simulink model "AccTarSel"  (R2018b)
settings: Solver=FixedStepDiscrete  StartTime=0.0  StopTime=inf  FixedStep=0.01  RelTol=1e-3
PostLoadFcn:
  | if any(exist('dsrtsu_mdlpostloadfcn', 'file') ~= 0), dsrtsu_mdlpostloadfcn('Execute', bdroot); end
values from neighbouring files (symbols this model uses):
  P_adtMaxBDC = 1.0    [AccTarSel.sldd]
  P_aFOCApproachIntpAcitve = -0.6    [AccTarSel.sldd]
  P_aFOCApproachIntpEnsure = -1.8    [AccTarSel.sldd]
  P_CutInEnable = 1.0    [AccTarSel.sldd]
  P_dAimMin = 4.5    [AccTarSel.sldd]
  P_dAimMinAVP = 1.5    [AccTarSel.sldd]
  P_dObjDrvOffMax = 5.0    [AccTarSel.sldd]
  P_dObjDrvOffMin = 3.0    [AccTarSel.sldd]
  P_dObjLowHystDecToStop = 4.5    [AccTarSel.sldd]
  P_dObjLowHystDecToStopAVP = 1.5    [AccTarSel.sldd]
  P_dObjUpperHystDecToStop = 5.0    [AccTarSel.sldd]
  P_dResMax = 5.0    [AccTarSel.sldd]
  P_dStandStill = 3.0    [AccTarSel.sldd]
  P_dStandStillMin = 2.0    [AccTarSel.sldd]
  P_dvarYMax4PO = 1.0    [AccTarSel.sldd]
  P_dyCutInThres = 3.6    [AccTarSel.sldd]
  P_facBDCInit = 0.7    [AccTarSel.sldd]
  P_facBDCIterCalc = 0.8    [AccTarSel.sldd]
  P_facFOCNegDiff = 0.3    [AccTarSel.sldd]
  P_facFOCPosDiff = 0.2    [AccTarSel.sldd]
  P_kapHystThres = 0.0005    [AccTarSel.sldd]
  P_PlausIntegDisable = 0.0    [AccTarSel.sldd]
  P_plausMin4PO = 0.5    [AccTarSel.sldd]
  P_probExistMin4PO = 0.8    [AccTarSel.sldd]
  P_StandObjEnable = 0.0    [AccTarSel.sldd]
  P_tAxTrackNegLower = 0.3    [AccTarSel.sldd]
  P_tAxTrackNegUpper = 0.6    [AccTarSel.sldd]
  P_tAxTrackPosLower = 1.0    [AccTarSel.sldd]
  P_tAxTrackPosUpper = 2.0    [AccTarSel.sldd]
  P_tBDCStartFilt = 0.2    [AccTarSel.sldd]
  P_tCSC = 3.5    [AccTarSel.sldd]
  P_tCurvFilt = 0.2    [AccTarSel.sldd]
  P_tCutInFilt = 0.5    [AccTarSel.sldd]
  P_tFiltAxAbsPONegFast = 0.1    [AccTarSel.sldd]
  P_tFiltAxAbsPONegSlow = 0.4    [AccTarSel.sldd]
  P_tFiltAxAbsPOPosFast = 1.2    [AccTarSel.sldd]
  P_tFiltAxAbsPOPosSlow = 2.0    [AccTarSel.sldd]
  P_tFiltAxAbsPOStand = 2.0    [AccTarSel.sldd]
  P_tFiltDAim = 0.1    [AccTarSel.sldd]
  P_tFiltDsd = 0.1    [AccTarSel.sldd]
  P_tFiltSpdLim = 3.0    [AccTarSel.sldd]
  P_tFiltVxAxPOFast = 0.15    [AccTarSel.sldd]
  P_tFiltVxAxPOSlow = 0.25    [AccTarSel.sldd]
  P_tFOCStatAccelFast = 4.0    [AccTarSel.sldd]
  P_tFOCStatAccelSlow = 3.5    [AccTarSel.sldd]
  P_tFOCStatDecelFast = 4.0    [AccTarSel.sldd]
  P_tFOCStatDecelSlow = 3.2    [AccTarSel.sldd]
  P_tMinDrvPhase = 2.0    [AccTarSel.sldd]
  P_tPredObjLeav = 1.2    [AccTarSel.sldd]
  P_tRollingFilt = 0.5    [AccTarSel.sldd]
  P_tRollingFinFilt = 1.0    [AccTarSel.sldd]
  P_tSSCNeg = 4.5    [AccTarSel.sldd]
  P_tSSCPos = 5.5    [AccTarSel.sldd]
  P_tToStop = 5.0    [AccTarSel.sldd]
  P_tToStopInBDC = 6.0    [AccTarSel.sldd]
  P_tToStopTrig = 4.0    [AccTarSel.sldd]
  P_vEgoDecToStop = 3.0    [AccTarSel.sldd]
  P_vEgoLowBDC = 4.0    [AccTarSel.sldd]
  P_vFOCNegDiff = 4.0    [AccTarSel.sldd]
  P_vFOCPosDiff = 5.0    [AccTarSel.sldd]
  P_vFOCStationaryFast = 15.0    [AccTarSel.sldd]
  P_vFOCStationarySlow = 5.0    [AccTarSel.sldd]
  P_vObjDrvOff = 0.5    [AccTarSel.sldd]
  P_vObjLowHystDecToStop = 0.5    [AccTarSel.sldd]
  P_vObjNoStop = 1.0    [AccTarSel.sldd]
  P_vObjReCalc = 1.0    [AccTarSel.sldd]
  P_vObjStop = 0.3    [AccTarSel.sldd]
  P_vObjUpperHystDecToStop = 0.8    [AccTarSel.sldd]
  P_vStandStill = 0.3    [AccTarSel.sldd]
  P_vStandStillHyst = 0.3    [AccTarSel.sldd]
  P_vyCutInThres = 0.5    [AccTarSel.sldd]
libraries: simulink x21, LPFilter x12
(part 7 of 11)

== system AccTarSel/ACC_Control/FollowObjCtrl/FollowObjValid/FOC_MIX ==
  aStat : Inport
  aApprh : Inport  Port=2
  tObjStop : Inport  Port=3
  FOCInfoK1 : Inport  Port=4
  SYS_Info_st : Inport  Port=5
  Bus Creator{,1..3} (4 alike) : BusCreator  Inputs=2
  Bus Selector : BusSelector  OutputSignals=dT
  Bus Selector1 : BusSelector  OutputSignals=FirstCyc,aFOC
  Constant : Constant  Value=3  OutDataTypeStr=single
  Constant1 : Constant  Value=0.1  OutDataTypeStr=single
  Constant2 : Constant  Value=0.4  OutDataTypeStr=single
  Constant4 : Constant  Value=5  OutDataTypeStr=single
  LPFilter : LPFilter/LPFilter  SystemSampleTime=-1
      settings: SourceProductName=CustomLib
  Lookup Table Dynamic : simulink/Lookup Tables/Lookup Table Dynamic  LookUpMeth=Interpolation-Use End Values  OutDataType=fixdt('single')  OutScaling=[]  OutputDataTypeScalingMode=Specify via dialog  OutDataTypeStr=single  DoSatur=off
      settings: SourceProductName=Simulink
  Lookup Table Dynamic1 : simulink/Lookup Tables/Lookup Table Dynamic  LookUpMeth=Interpolation-Use End Values  OutDataType=fixdt('single')  OutScaling=[]  OutputDataTypeScalingMode=Specify via dialog  OutDataTypeStr=single  DoSatur=off
      settings: SourceProductName=Simulink
  Min : MinMax  Inputs=2
  P_aFOCApproachIntpAcitve : Constant  Value=P_aFOCApproachIntpAcitve
  P_aFOCApproachIntpEnsure : Constant  Value=P_aFOCApproachIntpEnsure
  Subsystem : Subsystem
  Switch : Switch  Criteria=u2 > Threshold
  aFocMix : Outport
  wires:
  aApprh/1 -> Min/2, Subsystem/2(In2)
  Bus Creator/1 -> Lookup Table Dynamic/2
  aStat/1 -> Bus Creator1/2, Subsystem/1(In1), Min/1
  Bus Creator1/1 -> Lookup Table Dynamic/3
  P_aFOCApproachIntpEnsure/1 -> Bus Creator/1
  P_aFOCApproachIntpAcitve/1 -> Bus Creator/2
  Min/1 -> Bus Creator1/1, Lookup Table Dynamic/1
  Lookup Table Dynamic/1 -> LPFilter/1, Switch/1
  Switch/1 -> aFocMix/1
  LPFilter/1 -> Switch/3
  SYS_Info_st/1 -> Bus Selector/1
  Constant/1 -> Bus Creator2/1
  Constant4/1 -> Bus Creator2/2
  Constant2/1 -> Bus Creator3/1
  Bus Selector/1 -> LPFilter/2  "<dT>"
  tObjStop/1 -> Lookup Table Dynamic1/1
  Bus Creator2/1 -> Lookup Table Dynamic1/2
  Bus Creator3/1 -> Lookup Table Dynamic1/3
  Lookup Table Dynamic1/1 -> LPFilter/3
  FOCInfoK1/1 -> Bus Selector1/1
  Bus Selector1/1 -> Switch/2  "<FirstCyc>"
  Bus Selector1/2 -> LPFilter/4  "<aFOC>"
  Constant1/1 -> Bus Creator3/2

== system AccTarSel/ACC_Control/FollowObjCtrl/FollowObjValid/If Action Subsystem ==
  In1 : Inport
  Action Port : ActionPort  ActionType=then
  Out1 : Outport
  wires:
  In1/1 -> Out1/1

== system AccTarSel/ACC_Control/FollowObjCtrl/FollowObjValid/If Action Subsystem1 ==
  In1 : Inport
  Action Port : ActionPort  ActionType=else
  Out1 : Outport
  wires:
  In1/1 -> Out1/1

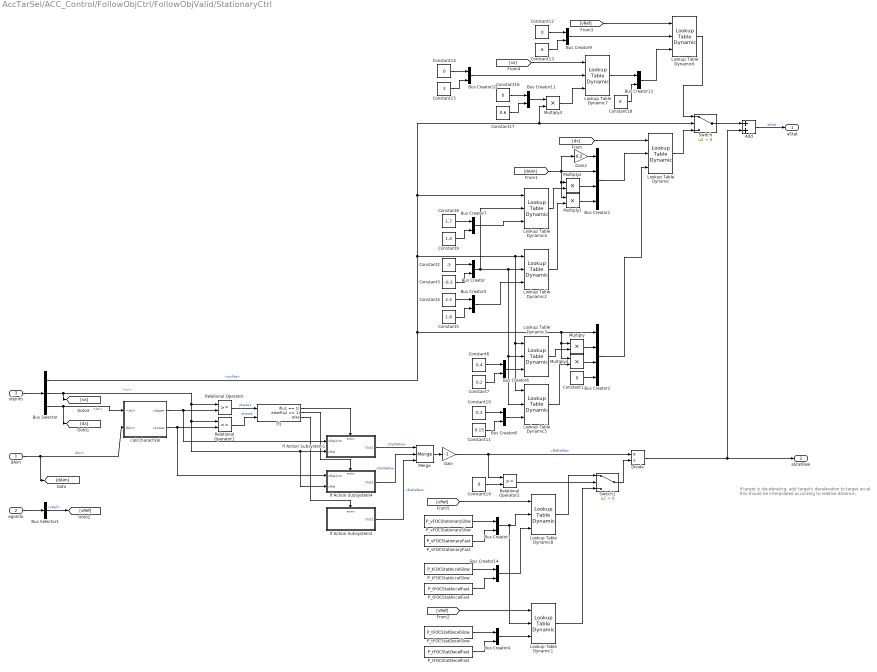
== system AccTarSel/ACC_Control/FollowObjCtrl/FollowObjValid/StationaryCtrl ==
  note: if target is decelerating, add target's deceleration to target accel.
      | this should be interpolated according to relative distance.
  dAim : Inport
  egoInfo : Inport  Port=2
  objInfo : Inport  Port=3
  Add : Sum
  Bus Creator{,3..12,14} (12 alike) : BusCreator  Inputs=2
  Bus Creator1 : BusCreator  Inputs=4
  Bus Creator2 : BusCreator  Inputs=4
  Bus Selector : BusSelector  OutputSignals=axAbs,vx,dx
  Bus Selector1 : BusSelector  OutputSignals=vRef
  Constant{1,12,14,16,18..19} (6 alike) : Constant  Value=0  OutDataTypeStr=single
  Constant10 : Constant  Value=0.3  OutDataTypeStr=single
  Constant11 : Constant  Value=0.15  OutDataTypeStr=single
  Constant13 : Constant  Value=6  OutDataTypeStr=single
  Constant15 : Constant  Value=3  OutDataTypeStr=single
  Constant17 : Constant  Value=0.6  OutDataTypeStr=single
  Constant2 : Constant  Value=-3  OutDataTypeStr=single
  Constant3 : Constant  Value=-0.3  OutDataTypeStr=single
  Constant4 : Constant  Value=2.5  OutDataTypeStr=single
  Constant5 : Constant  Value=1.8  OutDataTypeStr=single
  Constant6 : Constant  Value=0.4  OutDataTypeStr=single
  Constant7 : Constant  Value=0.2  OutDataTypeStr=single
  Constant8 : Constant  Value=1.7  OutDataTypeStr=single
  Constant9 : Constant  Value=1.4  OutDataTypeStr=single
  Divide : Product  Inputs=*/
  Gain : Gain  Gain=-1
  Gain2 : Gain  Gain=0.2
  If Action Subsystem1 : Subsystem  TreatAsAtomicUnit=on
  If Action Subsystem2 : Subsystem  TreatAsAtomicUnit=on
  If Action Subsystem4 : Subsystem  TreatAsAtomicUnit=on
  If1 : If  NumInputs=2  IfExpression=u1 == 1  ElseIfExpressions=u2 == 1
  Lookup Table Dynamic{,1..8} (9 alike) : simulink/Lookup Tables/Lookup Table Dynamic  LookUpMeth=Interpolation-Use End Values  OutDataType=fixdt('single')  OutScaling=[]  OutputDataTypeScalingMode=Specify via dialog  OutDataTypeStr=single  DoSatur=off
      settings: SourceProductName=Simulink
  Merge : Merge  Inputs=3
  Multiply{,1..4} (5 alike) : Product
  P_tFOCStatAccelFast : Constant  Value=P_tFOCStatAccelFast
  P_tFOCStatAccelSlow : Constant  Value=P_tFOCStatAccelSlow
  P_tFOCStatDecelFast : Constant  Value=P_tFOCStatDecelFast
  P_tFOCStatDecelSlow : Constant  Value=P_tFOCStatDecelSlow
  P_vFOCStationaryFast : Constant  Value=P_vFOCStationaryFast
  P_vFOCStationarySlow : Constant  Value=P_vFOCStationarySlow
  Relational Operator : RelationalOperator  OutDataTypeStr=boolean  RndMeth=Simplest
  Relational Operator1 : RelationalOperator  Operator=<=  OutDataTypeStr=boolean  RndMeth=Simplest
  Relational Operator2 : RelationalOperator  OutDataTypeStr=boolean  RndMeth=Simplest
  Switch : Switch  Criteria=u2 > Threshold
  Switch1 : Switch  Criteria=u2 > Threshold
  calcCharactVal : Subsystem
  aStat : Outport
  aStatRaw : Outport  Port=2
  wires:
  objInfo/1 -> Bus Selector/1
  Divide/1 -> Add/2, aStatRaw/1
  Merge/1 -> Gain/1
  dAim/1 -> [dAim], calcCharactVal/2(dAim)  "dAim"
  Bus Selector/3 -> [dx], calcCharactVal/1(<dx>)  "<dx>"
  Bus Selector/2 -> [vx], Relational Operator/1, If Action Subsystem1/2(vRel), If Action Subsystem4/2(vRel), Relational Operator1/1  "<vx>"
  calcCharactVal/2(vLower) -> If Action Subsystem4/1(vRelAim), Relational Operator1/2
  Relational Operator/1 -> If1/1  "phase1"
  Relational Operator1/1 -> If1/2  "phase2"
  If1/1 -> If Action Subsystem1/Action
  If1/2 -> If Action Subsystem4/Action
  If1/3 -> If Action Subsystem2/Action
  If Action Subsystem1/1(Out1) -> Merge/1  "vDeltaRaw"
  If Action Subsystem4/1(Out1) -> Merge/2  "vDeltaRaw"
  If Action Subsystem2/1(Out1) -> Merge/3  "vDeltaRaw"
  Bus Selector/1 -> Lookup Table Dynamic5/1, Lookup Table Dynamic3/1, Lookup Table Dynamic2/1, Lookup Table Dynamic4/1, Switch/2, Multiply3/2, Multiply4/1, Multiply/1, Bus Creator2/1  "<axAbs>"
  calcCharactVal/1(vUpper) -> If Action Subsystem1/1(vRelAim), Relational Operator/2
  Gain/1 -> Relational Operator2/1, Divide/1  "vDeltaRaw"
  [dx] -> Lookup Table Dynamic/1
  Gain2/1 -> Bus Creator1/1
  [dAim] -> Multiply2/1, Multiply1/1, Bus Creator1/2, Gain2/1
  Bus Creator2/1 -> Lookup Table Dynamic/3
  Bus Creator1/1 -> Lookup Table Dynamic/2
  egoInfo/1 -> Bus Selector1/1
  Bus Selector1/1 -> [vRef]  "<vRef>"
  [vRef] -> Lookup Table Dynamic1/1
  P_vFOCStationarySlow/1 -> Bus Creator3/1
  P_vFOCStationaryFast/1 -> Bus Creator3/2
  Bus Creator4/1 -> Lookup Table Dynamic1/3
  Switch/1 -> Add/1
  Add/1 -> aStat/1  "aStat"
  Multiply1/1 -> Bus Creator1/4
  Constant1/1 -> Bus Creator2/4
  Multiply/1 -> Bus Creator2/2
  Lookup Table Dynamic/1 -> Switch/3
  Constant2/1 -> Bus Creator/1
  Constant3/1 -> Bus Creator/2
  Constant5/1 -> Bus Creator5/2
  Constant4/1 -> Bus Creator5/1
  Bus Creator5/1 -> Lookup Table Dynamic2/3
  Bus Creator/1 -> Lookup Table Dynamic4/2, Lookup Table Dynamic5/2, Lookup Table Dynamic3/2, Lookup Table Dynamic2/2
  Lookup Table Dynamic2/1 -> Multiply1/2
  Constant6/1 -> Bus Creator6/1
  Constant7/1 -> Bus Creator6/2
  Bus Creator6/1 -> Lookup Table Dynamic3/3
  Lookup Table Dynamic3/1 -> Multiply/2
  P_tFOCStatDecelSlow/1 -> Bus Creator4/1
  P_tFOCStatDecelFast/1 -> Bus Creator4/2
  Bus Creator7/1 -> Lookup Table Dynamic4/3
  Constant8/1 -> Bus Creator7/1
  Constant9/1 -> Bus Creator7/2
  Lookup Table Dynamic4/1 -> Multiply2/2
  Multiply2/1 -> Bus Creator1/3
  Constant11/1 -> Bus Creator8/2
  Constant10/1 -> Bus Creator8/1
  Bus Creator8/1 -> Lookup Table Dynamic5/3
  [vRef] -> Lookup Table Dynamic6/1
  Bus Creator9/1 -> Lookup Table Dynamic6/2
  Constant13/1 -> Bus Creator9/2
  Constant12/1 -> Bus Creator9/1
  [vx] -> Lookup Table Dynamic7/1
  Constant14/1 -> Bus Creator10/1
  Constant15/1 -> Bus Creator10/2
  Bus Creator10/1 -> Lookup Table Dynamic7/2
  Bus Creator11/1 -> Multiply3/1
  Constant17/1 -> Bus Creator11/2
  Constant16/1 -> Bus Creator11/1
  Lookup Table Dynamic7/1 -> Bus Creator12/1
  Constant18/1 -> Bus Creator12/2
  Bus Creator12/1 -> Lookup Table Dynamic6/3
  Multiply3/1 -> Lookup Table Dynamic7/3
  Lookup Table Dynamic6/1 -> Switch/1
  Multiply4/1 -> Bus Creator2/3
  Lookup Table Dynamic5/1 -> Multiply4/2
  Constant19/1 -> Relational Operator2/2
  Relational Operator2/1 -> Switch1/2
  Switch1/1 -> Divide/2
  Lookup Table Dynamic8/1 -> Switch1/1
  P_tFOCStatAccelFast/1 -> Bus Creator14/2
  P_tFOCStatAccelSlow/1 -> Bus Creator14/1
  Bus Creator14/1 -> Lookup Table Dynamic8/3
  [vRef] -> Lookup Table Dynamic8/1
  Bus Creator3/1 -> Lookup Table Dynamic1/2, Lookup Table Dynamic8/2
  Lookup Table Dynamic1/1 -> Switch1/3

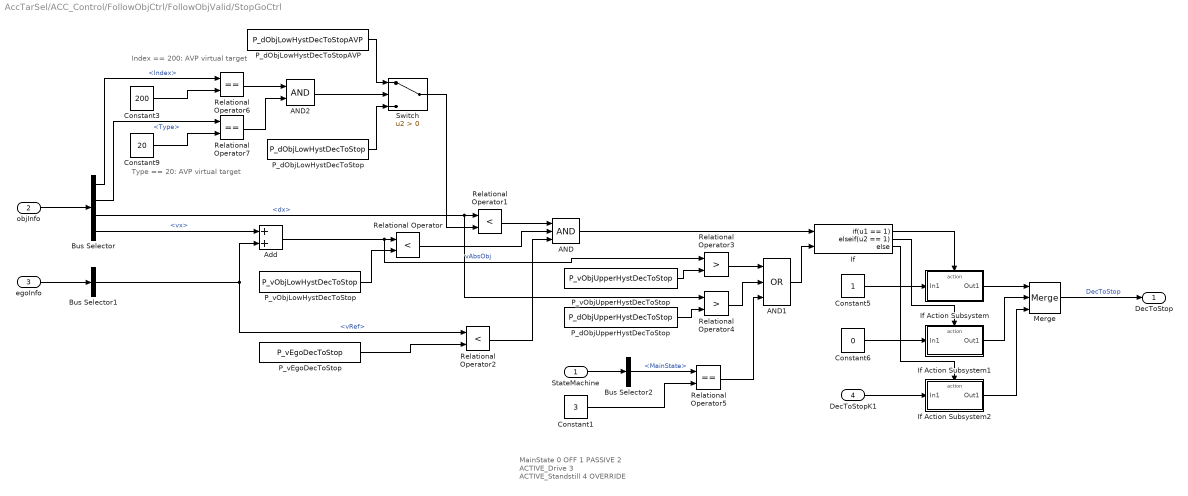
== system AccTarSel/ACC_Control/FollowObjCtrl/FollowObjValid/StopGoCtrl ==
  note: MainState
      | 0	OFF
      | 1	PASSIVE
      | 2	ACTIVE_Drive
      | 3	ACTIVE_Standstill
      | 4	OVERRIDE
  note: Type == 20: AVP virtual target
  note: Index == 200: AVP virtual target
  StateMachine : Inport
  objInfo : Inport  Port=2
  egoInfo : Inport  Port=3
  DecToStopK1 : Inport  Port=4
  AND : Logic  Inputs=3  AllPortsSameDT=off  OutDataTypeStr=boolean
  AND1 : Logic  Operator=OR  Inputs=3  AllPortsSameDT=off  OutDataTypeStr=boolean
  AND2 : Logic  AllPortsSameDT=off  OutDataTypeStr=boolean
  Add : Sum
  Bus Selector : BusSelector  OutputSignals=Index,Type,dx,vx
  Bus Selector1 : BusSelector  OutputSignals=vRef
  Bus Selector2 : BusSelector  OutputSignals=MainState
  Constant1 : Constant  Value=3  OutDataTypeStr=boolean
  Constant3 : Constant  Value=200  OutDataTypeStr=single
  Constant5 : Constant  OutDataTypeStr=boolean
  Constant6 : Constant  Value=0  OutDataTypeStr=boolean
  Constant9 : Constant  Value=20  OutDataTypeStr=single
  If : If  NumInputs=2  IfExpression=u1 == 1  ElseIfExpressions=u2 == 1
  If Action Subsystem : Subsystem  TreatAsAtomicUnit=on
  If Action Subsystem1 : Subsystem  TreatAsAtomicUnit=on
  If Action Subsystem2 : Subsystem  TreatAsAtomicUnit=on
  Merge : Merge  Inputs=3
  P_dObjLowHystDecToStop : Constant  Value=P_dObjLowHystDecToStop
  P_dObjLowHystDecToStopAVP : Constant  Value=P_dObjLowHystDecToStopAVP
  P_dObjUpperHystDecToStop : Constant  Value=P_dObjUpperHystDecToStop
  P_vEgoDecToStop : Constant  Value=P_vEgoDecToStop
  P_vObjLowHystDecToStop : Constant  Value=P_vObjLowHystDecToStop
  P_vObjUpperHystDecToStop : Constant  Value=P_vObjUpperHystDecToStop
  Relational Operator : RelationalOperator  Operator=<  OutDataTypeStr=boolean  RndMeth=Simplest
  Relational Operator1 : RelationalOperator  Operator=<  OutDataTypeStr=boolean  RndMeth=Simplest
  Relational Operator2 : RelationalOperator  Operator=<  OutDataTypeStr=boolean  RndMeth=Simplest
  Relational Operator3 : RelationalOperator  Operator=>  OutDataTypeStr=boolean  RndMeth=Simplest
  Relational Operator4 : RelationalOperator  Operator=>  OutDataTypeStr=boolean  RndMeth=Simplest
  Relational Operator5 : RelationalOperator  Operator===  OutDataTypeStr=boolean  RndMeth=Simplest
  Relational Operator6 : RelationalOperator  Operator===  OutDataTypeStr=boolean  RndMeth=Simplest
  Relational Operator7 : RelationalOperator  Operator===  OutDataTypeStr=boolean  RndMeth=Simplest
  Switch : Switch  Criteria=u2 > Threshold
  DecToStop : Outport
  wires:
  objInfo/1 -> Bus Selector/1
  egoInfo/1 -> Bus Selector1/1
  Bus Selector/4 -> Add/1  "<vx>"
  Bus Selector1/1 -> Relational Operator2/1, Add/2  "<vRef>"
  Add/1 -> Relational Operator3/1, Relational Operator/1  "vAbsObj"
  P_vObjLowHystDecToStop/1 -> Relational Operator/2
  Bus Selector/3 -> Relational Operator4/1, Relational Operator1/1  "<dx>"
  P_vEgoDecToStop/1 -> Relational Operator2/2
  Relational Operator1/1 -> AND/1
  Relational Operator/1 -> AND/2
  Relational Operator2/1 -> AND/3
  P_vObjUpperHystDecToStop/1 -> Relational Operator3/2
  P_dObjUpperHystDecToStop/1 -> Relational Operator4/2
  AND/1 -> If/1
  Relational Operator3/1 -> AND1/1
  Relational Operator4/1 -> AND1/2
  AND1/1 -> If/2
  If/1 -> If Action Subsystem/Action
  Constant5/1 -> If Action Subsystem/1(In1)
  If/2 -> If Action Subsystem1/Action
  Constant6/1 -> If Action Subsystem1/1(In1)
  If Action Subsystem/1(Out1) -> Merge/1
  If Action Subsystem1/1(Out1) -> Merge/2
  Merge/1 -> DecToStop/1  "DecToStop"
  If/3 -> If Action Subsystem2/Action
  DecToStopK1/1 -> If Action Subsystem2/1(In1)
  If Action Subsystem2/1(Out1) -> Merge/3
  StateMachine/1 -> Bus Selector2/1
  Bus Selector2/1 -> Relational Operator5/1  "<MainState>"
  Constant1/1 -> Relational Operator5/2
  Relational Operator5/1 -> AND1/3
  Bus Selector/1 -> Relational Operator6/1  "<Index>"
  Bus Selector/2 -> Relational Operator7/1  "<Type>"
  Relational Operator6/1 -> AND2/1
  Constant3/1 -> Relational Operator6/2
  Constant9/1 -> Relational Operator7/2
  Relational Operator7/1 -> AND2/2
  AND2/1 -> Switch/2
  P_dObjLowHystDecToStop/1 -> Switch/3
  P_dObjLowHystDecToStopAVP/1 -> Switch/1
  Switch/1 -> Relational Operator1/2

== system AccTarSel/ACC_Target_Selection/Subsystem/ValidObjCalc/CutInCalc ==
  objInfo : Inport
  dyToTraj : Inport  Port=2
  ATS_Internal_K1 : Inport  Port=3
  SYS_Info_st : Inport  Port=4
  Bus Selector : BusSelector  OutputSignals=Valid
  Constant1 : Constant  Value=0.5  OutDataTypeStr=single
  If Action Subsystem : Subsystem  TreatAsAtomicUnit=on
  If1 : If  IfExpression=u1 == 1
  Merge : Merge
  Merge1 : Merge
  Merge2 : Merge
  Relational Operator2 : RelationalOperator  Operator=>  OutDataTypeStr=boolean  RndMeth=Simplest
  Subsystem : Subsystem
  dyCutInPred : Outport
  probCutInFilt : Outport  Port=2
  isCutIn : Outport  Port=3
  probCutInRaw : Outport  Port=4
  wires:
  objInfo/1 -> Subsystem/1(objInfo), Bus Selector/1
  Constant1/1 -> Relational Operator2/2
  Relational Operator2/1 -> isCutIn/1  "isCutIn"
  If1/1 -> Subsystem/Action
  If1/2 -> If Action Subsystem/Action
  Subsystem/1(probCutInFilt) -> Merge/1
  If Action Subsystem/1(Out1) -> Merge/2
  Merge/1 -> probCutInFilt/1, Relational Operator2/1
  Subsystem/2(dyCutInPred) -> Merge1/1
  Merge1/1 -> dyCutInPred/1  "dyCutInPred"
  If Action Subsystem/2(Out2) -> Merge1/2
  dyToTraj/1 -> Subsystem/3(dyToTraj)
  Bus Selector/1 -> If1/1  "<Valid>"
  ATS_Internal_K1/1 -> Subsystem/2(ATS_Internal_K1)
  SYS_Info_st/1 -> Subsystem/4(SYS_Info_st)
  Merge2/1 -> probCutInRaw/1
  Subsystem/3(probCutInRaw) -> Merge2/1
  If Action Subsystem/3(Out3) -> Merge2/2

== system AccTarSel/ACC_Target_Selection/Subsystem/ValidObjCalc/EgoCourseDeviation ==
  objInfo : Inport
  egoTrajLane_st : Inport  Port=2
  Bus Selector : BusSelector  OutputSignals=Valid,dx,dy
  Constant : Constant  Value=0  OutDataTypeStr=single
  DistanceToTraj : Subsystem
  If : If  IfExpression=u1 == 1
  If Action Subsystem : Subsystem  TreatAsAtomicUnit=on
  Merge : Merge
  dyToTraj : Outport
  wires:
  Bus Selector/3 -> DistanceToTraj/2(In2)  "<dy>"
  Bus Selector/2 -> DistanceToTraj/1(In1)  "<dx>"
  egoTrajLane_st/1 -> DistanceToTraj/3(In3)
  objInfo/1 -> Bus Selector/1
  Bus Selector/1 -> If/1  "<Valid>"
  If/1 -> DistanceToTraj/Action
  If/2 -> If Action Subsystem/Action
  Constant/1 -> If Action Subsystem/1(In1)
  DistanceToTraj/1(Out1) -> Merge/1
  If Action Subsystem/1(Out1) -> Merge/2
  Merge/1 -> dyToTraj/1  "dyToTraj"

== system AccTarSel/ACC_Target_Selection/Subsystem/ValidObjCalc/LanePlausCalc ==
  note: logic to be expanded:
      | 1. plausibility should be independently calculated for each lane(left, ego and right)
      | 2. plausibility of each lane should be integrated according to coresponding probability
  probEgoLane : Inport
  isCutIn : Inport  Port=2
  objInfo : Inport  Port=3
  ATS_Internal_K1 : Inport  Port=4
  SYS_Info_st : Inport  Port=5
  Add : Sum
  Bus Selector : BusSelector  OutputSignals=ID,plausEgoLane
  Bus Selector1 : BusSelector  OutputSignals=dT
  Bus Selector2 : BusSelector  OutputSignals=ID
  Constant : Constant  Value=0.6  OutDataTypeStr=single
  Constant1 : Constant  OutDataTypeStr=single
  Constant2 : Constant  Value=0  OutDataTypeStr=single
  Constant3 : Constant  Value=0  OutDataTypeStr=single
  Constant4 : Constant  Value=P_PlausIntegDisable  OutDataTypeStr=boolean
  If : If  IfExpression=u1 == 1
  If Action Subsystem : Subsystem  TreatAsAtomicUnit=on
  If Action Subsystem1 : Subsystem  TreatAsAtomicUnit=on
  Max : MinMax  Function=max  Inputs=2
  Merge : Merge
  Min : MinMax  Inputs=2
  Min1 : MinMax  Function=max  Inputs=2
  Multiply : Product
  Relational Operator : RelationalOperator  Operator=~=  OutDataTypeStr=boolean  RndMeth=Simplest
  Switch : Switch  Criteria=u2 > Threshold
  Switch1 : Switch  Criteria=u2 > Threshold
  Out1 : Outport
  wires:
  isCutIn/1 -> If/1
  If/1 -> If Action Subsystem/Action
  probEgoLane/1 -> Multiply/1, Switch1/1
  If/2 -> If Action Subsystem1/Action
  If Action Subsystem/1(Out1) -> Merge/1
  If Action Subsystem1/1(Out1) -> Merge/2
  Merge/1 -> Out1/1
  Max/1 -> If Action Subsystem/1(In1)
  Constant/1 -> Max/1
  ATS_Internal_K1/1 -> Bus Selector/1
  Multiply/1 -> Add/1
  Add/1 -> Min/1
  Constant1/1 -> Min/2
  Min/1 -> Min1/1
  Constant2/1 -> Min1/2
  SYS_Info_st/1 -> Bus Selector1/1
  Bus Selector1/1 -> Multiply/2  "<dT>"
  objInfo/1 -> Bus Selector2/1
  Bus Selector2/1 -> Relational Operator/1  "<ID>"
  Bus Selector/1 -> Relational Operator/2  "<ID>"
  Relational Operator/1 -> Switch/2
  Constant3/1 -> Switch/1
  Bus Selector/2 -> Switch/3  "<plausEgoLane>"
  Switch/1 -> Add/2
  Constant4/1 -> Switch1/2
  Min1/1 -> Switch1/3
  Switch1/1 -> Max/2, If Action Subsystem1/1(In1)

== system AccTarSel/ACC_Target_Selection/Subsystem/ValidObjCalc/LaneProbCalc ==
  objInfo : Inport
  In2 : Inport  Port=2
  ATS_Internal_K1 : Inport  Port=3
  Bus Selector : BusSelector  OutputSignals=Valid,dx,ID
  Constant : Constant  Value=0  OutDataTypeStr=single
  If : If  IfExpression=u1 == 1
  If Action Subsystem : Subsystem  TreatAsAtomicUnit=on
  Merge : Merge
  Subsystem : Subsystem
  Out1 : Outport
  wires:
  objInfo/1 -> Bus Selector/1
  Bus Selector/1 -> If/1  "<Valid>"
  If/1 -> Subsystem/Action
  In2/1 -> Subsystem/3(In2)
  If/2 -> If Action Subsystem/Action
  Constant/1 -> If Action Subsystem/1(In1)
  Subsystem/1(probEgoTraj) -> Merge/1
  If Action Subsystem/1(Out1) -> Merge/2
  Merge/1 -> Out1/1
  ATS_Internal_K1/1 -> Subsystem/4(ATS_Internal_K1)
  Bus Selector/2 -> Subsystem/1(<dx>)  "<dx>"
  Bus Selector/3 -> Subsystem/2(ID)  "<ID>"
